simulink model "ThreephaseInverter"  (R2016a)
settings: Solver=VariableStepAuto  StartTime=0.0  StopTime=0.8  RelTol=1e-3
libraries: powerlib x20, powerlib_meascontrol x1
settings Model: Creator=enes_  LastModifiedBy=enes_

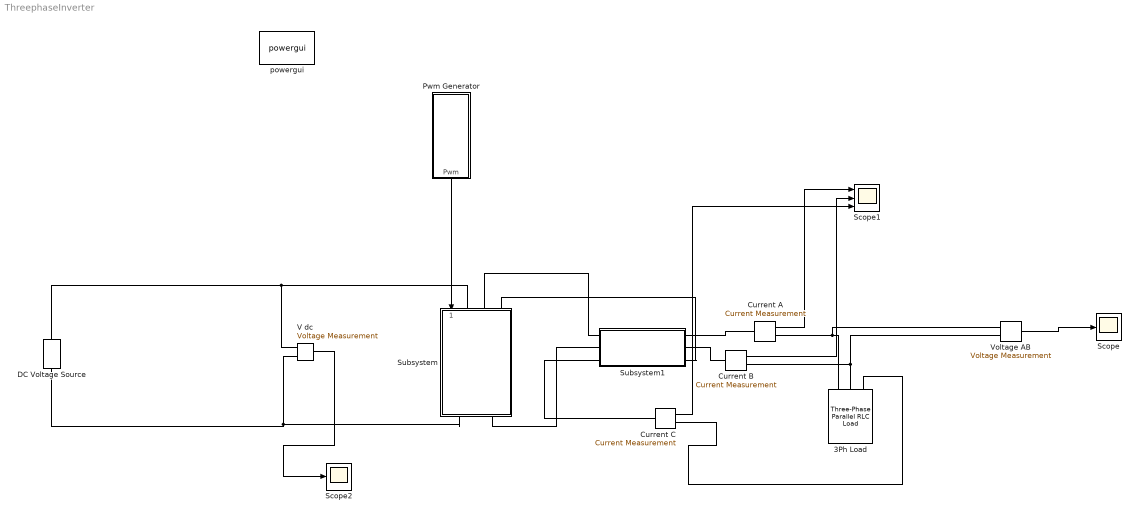
== system ThreephaseInverter ==
  "3Ph Load " : powerlib/Elements/Three-Phase Parallel RLC Load  LConnTagsString=A|B|C  Configuration=Y (floating)  NominalVoltage=415  Vabc=[1e3 1e3 1e3]  Vabcp=[1e3 1e3 1e3]  NominalFrequency=50  UnbalancedPower=off  ActivePower=5e3  InductivePower=0  CapacitivePower=0  Pabc=[10e3 9e3 11e3]  QLabc=[100 90 110]  QCabc=[100 90 110]  Pabcp=[10e3 9e3 11e3]  QLabcp=[100 90 110]  QCabcp=[100 90 110]  Measurements=None  LoadType=constant Z
  Current A : powerlib/Measurements/Current Measurement  PhasorSimulation=off  OutputType=Complex  PSBequivalent=0
  Current B : powerlib/Measurements/Current Measurement  PhasorSimulation=off  OutputType=Complex  PSBequivalent=0
  Current C : powerlib/Measurements/Current Measurement  PhasorSimulation=off  OutputType=Complex  PSBequivalent=0
  DC Voltage Source : powerlib/Electrical Sources/DC Voltage Source  Amplitude=415*2*sqrt(2/3)  Measurements=None
  Pwm Generator : Subsystem
  Scope : Scope
  Scope1 : Scope  NumInputPorts=3
  Scope2 : Scope
  Subsystem : Subsystem
  Subsystem1 : Subsystem
  "V dc " : powerlib/Measurements/Voltage Measurement  PhasorSimulation=off  OutputType=Complex  PSBequivalent=0
  Voltage AB : powerlib/Measurements/Voltage Measurement  PhasorSimulation=off  OutputType=Complex  PSBequivalent=0
  powergui : powerlib/powergui  Priority=1  SimulationMode=Continuous  SolverType=Tustin  SampleTime=50e-6  frequency=60  SPID=on  DisableSnubberDevices=off  DisableRonSwitches=off  DisableVfSwitches=off  SwTol=0  DisplayEquations=off  Interpol=off  ExternalGateDelay=off  methode=off  Ts=10  FunctionMessages=off  echomessages=off  HookPort=off  EnableUseOfTLC=off  x0status=blocks  frequencyindice=0  Pbase=100e6  ErrMax=1e-4  Iterations=50  UnitsV=kV  UnitsW=MW  buscounter=0  RestoreLinks=warning  ResistiveCurrentMeasurement=off  Frange=[0:2:500]  Ylog=off  Xlog=on  ShowGrid=off  save=off  variable=ZData  structure=ScopeData2  ZoomFFT=off  StartTime=0.6  cycles=4  DisplayStyle=4  fundamental=50  FreqAxis=on  MaxFrequency=650  frequencyindicesteady=1  RmsSteady=1  display=off
  wires:
  "V dc "/1 -> Scope2/1
  Pwm Generator/1(Pwm) -> Subsystem/1(PWM)
  Voltage AB/1 -> Scope/1
  Current A/1 -> Scope1/1
  Current B/1 -> Scope1/2
  Current C/1 -> Scope1/3
  connections:
  "V dc "/LConn2 -- Subsystem/RConn1 -- DC Voltage Source/LConn1
  "V dc "/LConn1 -- DC Voltage Source/RConn1 -- Subsystem/LConn1
  Subsystem1/LConn1 -- Subsystem/LConn2
  Subsystem1/LConn2 -- Subsystem/RConn2
  Subsystem1/RConn3 -- Subsystem/LConn3
  "3Ph Load "/LConn1 -- Current A/RConn1 -- Voltage AB/LConn1
  Voltage AB/LConn2 -- "3Ph Load "/LConn2 -- Current B/RConn1
  Current A/LConn1 -- Subsystem1/RConn1
  Current B/LConn1 -- Subsystem1/RConn2
  Subsystem1/LConn3 -- Current C/LConn1
  Current C/RConn1 -- "3Ph Load "/LConn3

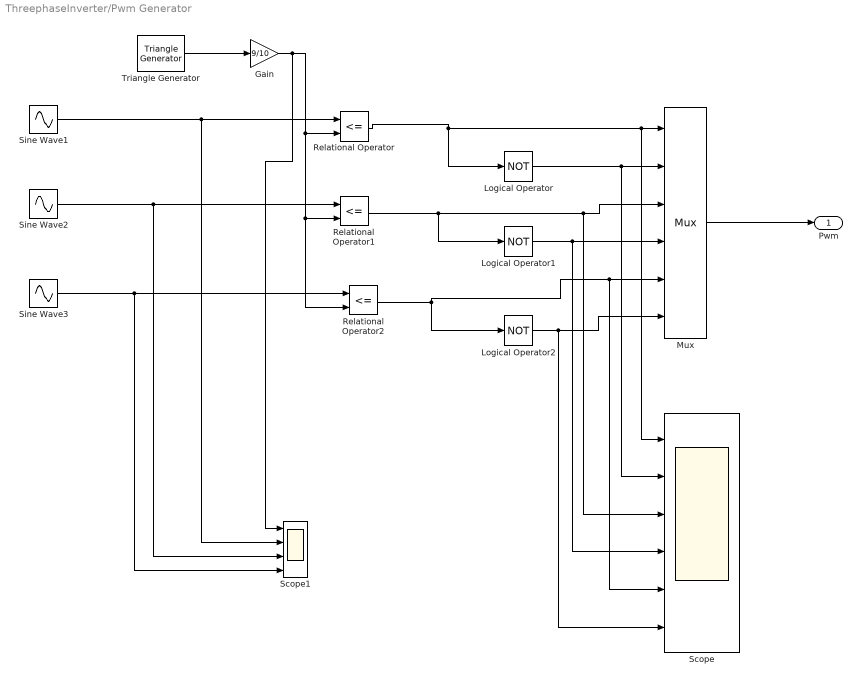
== system ThreephaseInverter/Pwm Generator ==
  Gain : Gain  Gain=9/10
  Logical Operator : Logic  Operator=NOT  AllPortsSameDT=off  OutDataTypeStr=boolean
  Logical Operator1 : Logic  Operator=NOT  AllPortsSameDT=off  OutDataTypeStr=boolean
  Logical Operator2 : Logic  Operator=NOT  AllPortsSameDT=off  OutDataTypeStr=boolean
  Mux : Mux  Inputs=6
  Relational Operator : RelationalOperator  Operator=<=  OutDataTypeStr=boolean
  Relational Operator1 : RelationalOperator  Operator=<=  OutDataTypeStr=boolean
  Relational Operator2 : RelationalOperator  Operator=<=  OutDataTypeStr=boolean
  Scope : Scope  NumInputPorts=6
  Scope1 : Scope  NumInputPorts=4
  Sine Wave1 : Sin  Frequency=50*2*pi  SampleTime=0
  Sine Wave2 : Sin  Frequency=50*2*pi  Phase=2*pi/3  SampleTime=0
  Sine Wave3 : Sin  Frequency=50*2*pi  Phase=4*pi/3  SampleTime=0
  Triangle Generator : powerlib_meascontrol/Pulse & Signal Generators/Triangle Generator  Freq=1000  Phase=0  Ts=0
  Pwm : Outport
  wires:
  Triangle Generator/1 -> Gain/1
  Sine Wave1/1 -> Scope1/2, Relational Operator/1
  Sine Wave3/1 -> Scope1/4, Relational Operator2/1
  Gain/1 -> Scope1/1, Relational Operator2/2, Relational Operator1/2, Relational Operator/2
  Relational Operator/1 -> Scope/1, Mux/1, Logical Operator/1
  Relational Operator1/1 -> Scope/3, Mux/3, Logical Operator1/1
  Relational Operator2/1 -> Scope/5, Mux/5, Logical Operator2/1
  Logical Operator2/1 -> Scope/6, Mux/6
  Logical Operator1/1 -> Scope/4, Mux/4
  Logical Operator/1 -> Scope/2, Mux/2
  Mux/1 -> Pwm/1
  Sine Wave2/1 -> Scope1/3, Relational Operator1/1

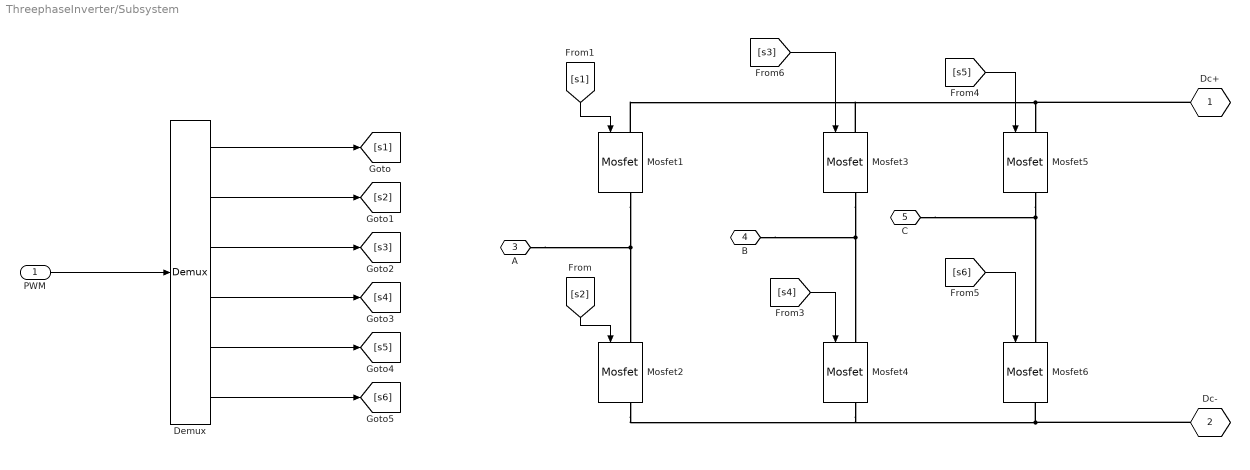
== system ThreephaseInverter/Subsystem ==
  PWM : Inport
  Demux : Demux  Outputs=6
  Mosfet{1..6} (6 alike) : powerlib/Power Electronics/Mosfet  Ron=0.1  Lon=0  Rd=0.01  Vfd=0  IC=0  Rs=1e5  Cs=inf  Measurements=on
  Dc+ : PMIOPort  Tag=PMCPort  Port=1  Side=Left
  Dc- : PMIOPort  Tag=PMCPort  Port=2  Side=Right
  A : PMIOPort  Port=3  Side=Left
  B : PMIOPort  Port=4  Side=Right
  C : PMIOPort  Port=5  Side=Left
  wires:
  Demux/1 -> [s1]
  Demux/2 -> [s2]
  Demux/3 -> [s3]
  Demux/4 -> [s4]
  Demux/5 -> [s5]
  Demux/6 -> [s6]
  [s1] -> Mosfet1/1
  [s2] -> Mosfet2/1
  [s3] -> Mosfet3/1
  [s4] -> Mosfet4/1
  [s5] -> Mosfet5/1
  [s6] -> Mosfet6/1
  PWM/1 -> Demux/1
  connections:
  Mosfet1/RConn1 -- A/RConn1 -- Mosfet2/LConn1
  Mosfet3/RConn1 -- B/RConn1 -- Mosfet4/LConn1
  Mosfet5/RConn1 -- Mosfet6/LConn1 -- C/RConn1
  Dc+/RConn1 -- Mosfet1/LConn1 -- Mosfet3/LConn1 -- Mosfet5/LConn1
  Dc-/RConn1 -- Mosfet2/RConn1 -- Mosfet4/RConn1 -- Mosfet6/RConn1

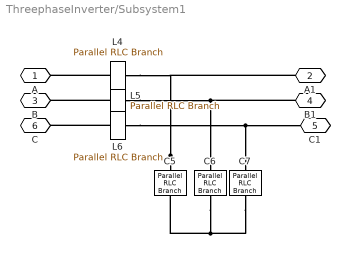
== system ThreephaseInverter/Subsystem1 ==
  C5 : powerlib/Elements/Parallel RLC Branch  LConnTagsString=a  RConnTagsString=__new0  BranchType=C  Resistance=inf  Inductance=inf  SetiL0=off  InitialCurrent=0  Capacitance=20e-6  Setx0=off  InitialVoltage=0  Measurements=None
  C6 : powerlib/Elements/Parallel RLC Branch  LConnTagsString=a  RConnTagsString=__new0  BranchType=C  Resistance=inf  Inductance=inf  SetiL0=off  InitialCurrent=0  Capacitance=20e-6  Setx0=off  InitialVoltage=0  Measurements=None
  C7 : powerlib/Elements/Parallel RLC Branch  LConnTagsString=a  RConnTagsString=__new0  BranchType=C  Resistance=inf  Inductance=inf  SetiL0=off  InitialCurrent=0  Capacitance=20e-6  Setx0=off  InitialVoltage=0  Measurements=None
  L4 : powerlib/Elements/Parallel RLC Branch  LConnTagsString=a  RConnTagsString=__new0  BranchType=L  Resistance=inf  Inductance=10-3  SetiL0=off  InitialCurrent=0  Capacitance=1.3e-3  Setx0=off  InitialVoltage=0  Measurements=None
  L5 : powerlib/Elements/Parallel RLC Branch  LConnTagsString=a  RConnTagsString=__new0  BranchType=L  Resistance=inf  Inductance=10e-3  SetiL0=off  InitialCurrent=0  Capacitance=1.3e-3  Setx0=off  InitialVoltage=0  Measurements=None
  L6 : powerlib/Elements/Parallel RLC Branch  LConnTagsString=a  RConnTagsString=__new0  BranchType=L  Resistance=inf  Inductance=10e-3  SetiL0=off  InitialCurrent=0  Capacitance=1.3e-3  Setx0=off  InitialVoltage=0  Measurements=None
  A : PMIOPort  Port=1  Side=Left
  A1 : PMIOPort  Port=2  Side=Right
  B : PMIOPort  Port=3  Side=Left
  B1 : PMIOPort  Port=4  Side=Right
  C1 : PMIOPort  Port=5  Side=Left
  C : PMIOPort  Port=6  Side=Right
  connections:
  C6/RConn1 -- C5/RConn1 -- C7/RConn1
  L5/RConn1 -- C6/LConn1 -- B1/RConn1
  C5/LConn1 -- L4/RConn1 -- A1/RConn1
  L6/RConn1 -- C7/LConn1 -- C1/RConn1
  L4/LConn1 -- A/RConn1
  L5/LConn1 -- B/RConn1
  L6/LConn1 -- C/RConn1
